simulink model "A320_Model_v1_4_3"  (R2016b)
settings: Solver=ode4  StartTime=0.0  StopTime=500  FixedStep=0.01  RelTol=1e-3
values from neighbouring files (symbols this model uses):
  er_enable = 0    [Initialization_v1_4_3.m]
  Initial_angular_rates = [0 0 0]    [Initialization_v1_4_3.m]
  initial_euler_angles = [Euler_roll_init Euler_pitch_init Euler_yaw_init]*180/pi    [Initialization_v1_4_3.m]
  initial_mulh = [41.108891 29.021111 9000]    [Initialization_v1_4_3.m]
  initial_vel_NED = transpose(DCM_init)*[U_init ; V_init ; W_init]    [Initialization_v1_4_3.m]
  tr_enable = 0    [Initialization_v1_4_3.m]
  trim_enable = 1    [Initialization_v1_4_3.m]
undefined symbols (not defined in the file or in its folder): a_Earth, acc_rand_samp, acc_rand_var, act_ang_lim_1, act_ang_lim_2, act_ang_lim_3, act_ang_lim_4, act_rate_lim_1, act_rate_lim_2, act_rate_lim_3, act_rate_lim_4, aero_CD0, aero_CD_beta, aero_CD_del_e, aero_Cl_del_a, aero_CL_del_e, aero_Cl_del_r, aero_Cl_r, aero_Cm_alpha, aero_Cm_alpha_dot, aero_Cm_del_e, aero_Cm_q, aero_Cn_beta, aero_Cn_del_r, aero_Cn_r, aero_lt_alpha_flap_CD, aero_lt_alpha_flap_CL, aero_lt_alpha_for_CD, aero_lt_alpha_for_CL, aero_lt_beta_Cl0, aero_lt_beta_CY, aero_lt_beta_for_Cl0, aero_lt_beta_for_CY, aero_lt_flap_Cm0, aero_lt_flap_for_CD, aero_lt_flap_for_CL, aero_lt_flap_for_Cm0, air_density_at_surface, air_pressure_at_surface, Aircraft_initial_mass, Aircraft_mean_chord, Aircraft_referance_area, Aircraft_wingspan, del_a_trimmed, del_e_trimmed, del_f_trimmed, del_r_trimmed, del_t_trimmed, e_Earth, engine_lt_h_for_Thrust, engine_lt_h_M_Thrust, engine_lt_M_for_Thrust, engine_number, gas_constant, gyro_rand_samp, gyro_rand_var, heat_ratio, Inertial_matrix, lapse_rate, max_thrust ... (+8)
libraries: simulink x2, aerolibtransform2 x1
settings Model: Creator=Nazmi  LastModifiedBy=Nazmi

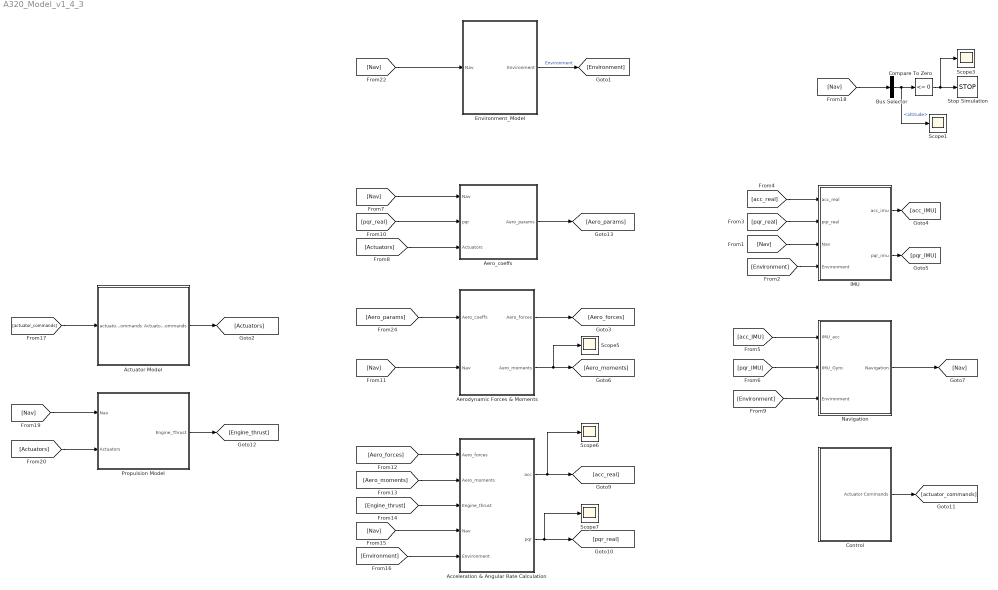
== system A320_Model_v1_4_3 ==
  Acceleration & Angular Rate Calculation : Subsystem
  Actuator Model : Subsystem
  Aero_coeffs : Subsystem
  Aerodynamic Forces & Moments : Subsystem
  Bus Selector : BusSelector  OutputSignals=mulh.altitude
  Compare To Zero : simulink/Logic and Bit Operations/Compare To Zero  relop=<=  OutDataTypeStr=boolean
  Control : Subsystem
  Environment_Model : Subsystem
  IMU : Subsystem
  Navigation : Subsystem
  "Propulsion Model " : Subsystem
  Scope{1,3,5..7} (5 alike) : Scope
  Stop Simulation : Stop
  wires:
  Navigation/1(Navigation) -> [Nav]
  [acc_IMU] -> Navigation/1(IMU_acc)
  [pqr_IMU] -> Navigation/2(IMU_Gyro)
  [Nav] -> Environment_Model/1(Nav)
  Environment_Model/1(Environment) -> [Environment]  "Environment"
  [acc_real] -> IMU/1(acc_real)
  [pqr_real] -> IMU/2(pqr_real)
  [Nav] -> IMU/3(Nav)
  [Environment] -> IMU/4(Environment)
  IMU/1(acc_imu) -> [acc_IMU]
  IMU/2(pqr_imu) -> [pqr_IMU]
  Aero_coeffs/1(Aero_params) -> [Aero_params]
  Actuator Model/1(Actuator_Commands) -> [Actuators]
  [Nav] -> Aero_coeffs/1(Nav)
  [Actuators] -> Aero_coeffs/3(Actuators)
  [Environment] -> Navigation/3(Environment)
  [pqr_real] -> Aero_coeffs/2(pqr)
  [Aero_params] -> Aerodynamic Forces & Moments/1(Aero_coeffs)
  [Nav] -> Aerodynamic Forces & Moments/2(Nav)
  Aerodynamic Forces & Moments/1(Aero_forces) -> [Aero_forces]
  Aerodynamic Forces & Moments/2(Aero_moments) -> [Aero_moments], Scope5/1
  [Aero_forces] -> Acceleration & Angular Rate Calculation/1(Aero_forces)
  [Aero_moments] -> Acceleration & Angular Rate Calculation/2(Aero_moments)
  [Engine_thrust] -> Acceleration & Angular Rate Calculation/3(Engine_thrust)
  [Nav] -> Acceleration & Angular Rate Calculation/4(Nav)
  [Environment] -> Acceleration & Angular Rate Calculation/5(Environment)
  Acceleration & Angular Rate Calculation/1(acc) -> [acc_real], Scope6/1
  Acceleration & Angular Rate Calculation/2(pqr) -> [pqr_real], Scope7/1
  Control/1(Actuator Commands) -> [actuator_commands]
  [actuator_commands] -> Actuator Model/1(actuator_commands)
  [Nav] -> Bus Selector/1
  Bus Selector/1 -> Compare To Zero/1, Scope1/1  "<altitude>"
  Compare To Zero/1 -> Stop Simulation/1, Scope3/1
  [Nav] -> "Propulsion Model "/1(Nav)
  [Actuators] -> "Propulsion Model "/2(Actuators)
  "Propulsion Model "/1("Engine_Thrust ") -> [Engine_thrust]

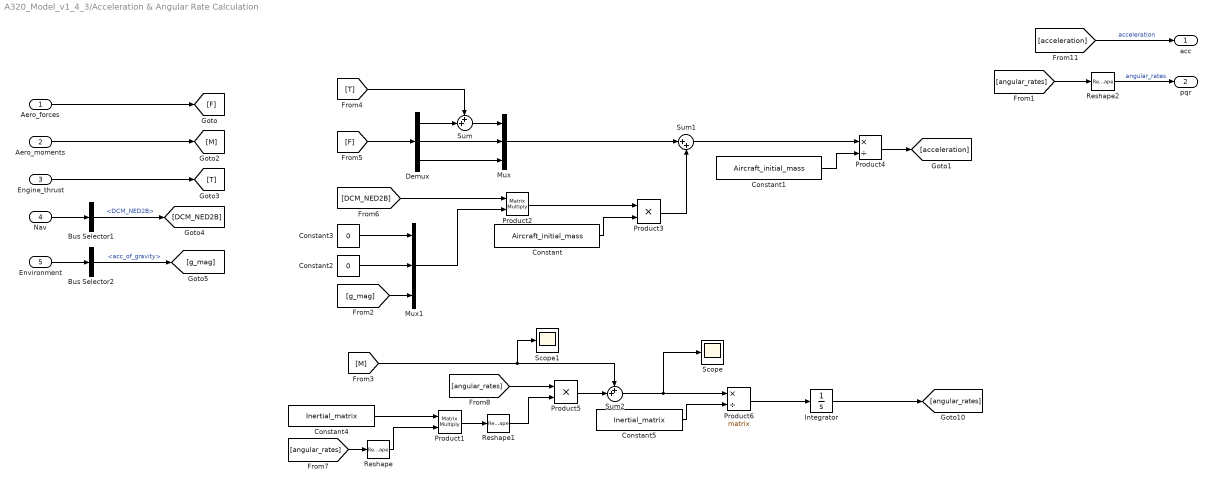
== system A320_Model_v1_4_3/Acceleration & Angular Rate Calculation ==
  Aero_forces : Inport
  Aero_moments : Inport  Port=2
  Engine_thrust : Inport  Port=3
  Nav : Inport  Port=4
  Environment : Inport  Port=5
  Bus Selector1 : BusSelector  OutputSignals=DCM_NED2B
  Bus Selector2 : BusSelector  OutputSignals=acc_of_gravity
  Constant : Constant  Value=Aircraft_initial_mass
  Constant1 : Constant  Value=Aircraft_initial_mass
  Constant2 : Constant  Value=0
  Constant3 : Constant  Value=0
  Constant4 : Constant  Value=Inertial_matrix
  Constant5 : Constant  Value=Inertial_matrix
  Demux : Demux  Outputs=3
  Integrator : Integrator  InitialCondition=Initial_angular_rates
  Mux : Mux  Inputs=3
  Mux1 : Mux  Inputs=3
  Product1 : Product  Multiplication=Matrix(*)  RndMeth=Zero
  Product2 : Product  Multiplication=Matrix(*)  RndMeth=Zero
  Product3 : Product  RndMeth=Zero
  Product4 : Product  Inputs=*/  RndMeth=Zero
  Product5 : Product  RndMeth=Zero
  Product6 : Product  Inputs=*/  Multiplication=Matrix(*)  RndMeth=Zero
  Reshape : Reshape  OutputDimensionality=Column vector (2-D)
  Reshape1 : Reshape  OutputDimensionality=Row vector (2-D)
  Reshape2 : Reshape
  Scope : Scope
  Scope1 : Scope
  Sum : Sum  Inputs=++|
  Sum1 : Sum  Inputs=|++
  Sum2 : Sum  Inputs=++|
  acc : Outport
  pqr : Outport  Port=2
  wires:
  [acceleration] -> acc/1  "acceleration"
  Aero_forces/1 -> [F]
  Aero_moments/1 -> [M]
  Engine_thrust/1 -> [T]
  Nav/1 -> Bus Selector1/1
  Environment/1 -> Bus Selector2/1
  Bus Selector1/1 -> [DCM_NED2B]  "<DCM_NED2B>"
  Bus Selector2/1 -> [g_mag]  "<acc_of_gravity>"
  Demux/1 -> Sum/2
  Sum/1 -> Mux/1
  [T] -> Sum/1
  Demux/2 -> Mux/2
  Demux/3 -> Mux/3
  [F] -> Demux/1
  [DCM_NED2B] -> Product2/1
  Product2/1 -> Product3/1
  Constant/1 -> Product3/2
  Mux/1 -> Sum1/1
  Product3/1 -> Sum1/2
  Sum1/1 -> Product4/1
  Constant1/1 -> Product4/2
  Product4/1 -> [acceleration]
  [g_mag] -> Mux1/3
  Constant3/1 -> Mux1/1
  Constant2/1 -> Mux1/2
  Mux1/1 -> Product2/2
  Product6/1 -> Integrator/1
  Constant5/1 -> Product6/2
  Sum2/1 -> Product6/1, Scope/1
  Product5/1 -> Sum2/2
  [M] -> Sum2/1, Scope1/1
  [angular_rates] -> Product5/1
  [angular_rates] -> Reshape/1
  Constant4/1 -> Product1/1
  Integrator/1 -> [angular_rates]
  Product1/1 -> Reshape1/1
  Reshape1/1 -> Product5/2
  Reshape/1 -> Product1/2
  [angular_rates] -> Reshape2/1
  Reshape2/1 -> pqr/1  "angular_rates"

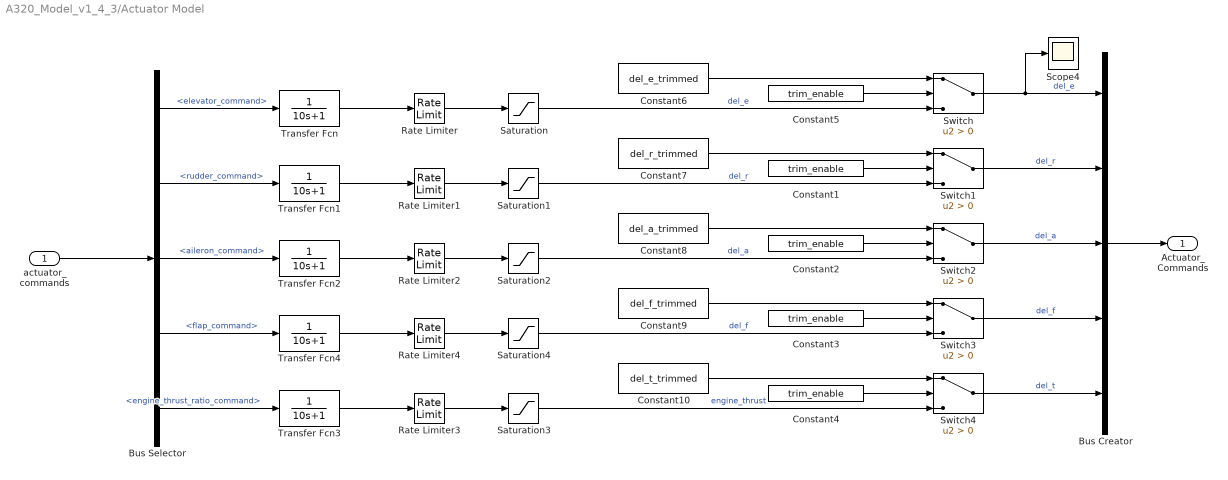
== system A320_Model_v1_4_3/Actuator Model ==
  actuator_commands : Inport
  Bus Creator : BusCreator  Inputs=5
  Bus Selector : BusSelector  OutputSignals=elevator_command,rudder_command,aileron_command,flap_command,engine_thrust_ratio_command
  Constant{1..5} (5 alike) : Constant  Value=trim_enable
  Constant10 : Constant  Value=del_t_trimmed
  Constant6 : Constant  Value=del_e_trimmed
  Constant7 : Constant  Value=del_r_trimmed
  Constant8 : Constant  Value=del_a_trimmed
  Constant9 : Constant  Value=del_f_trimmed
  Rate Limiter : RateLimiter  RisingSlewLimit=act_rate_lim_1  FallingSlewLimit=-act_rate_lim_1  SampleTimeMode=inherited
  Rate Limiter1 : RateLimiter  RisingSlewLimit=act_rate_lim_2  FallingSlewLimit=-act_rate_lim_2  SampleTimeMode=inherited
  Rate Limiter2 : RateLimiter  RisingSlewLimit=act_rate_lim_3  FallingSlewLimit=-act_rate_lim_3  SampleTimeMode=inherited
  Rate Limiter3 : RateLimiter  RisingSlewLimit=act_rate_lim_4  FallingSlewLimit=-act_rate_lim_4  SampleTimeMode=inherited
  Rate Limiter4 : RateLimiter  RisingSlewLimit=act_rate_lim_3  FallingSlewLimit=-act_rate_lim_3  SampleTimeMode=inherited
  Saturation : Saturate  UpperLimit=act_ang_lim_1  LowerLimit=-act_ang_lim_1
  Saturation1 : Saturate  UpperLimit=act_ang_lim_2  LowerLimit=-act_ang_lim_2
  Saturation2 : Saturate  UpperLimit=act_ang_lim_3  LowerLimit=-act_ang_lim_3
  Saturation3 : Saturate  UpperLimit=act_ang_lim_4  LowerLimit=0
  Saturation4 : Saturate  UpperLimit=act_ang_lim_3  LowerLimit=-act_ang_lim_3
  Scope4 : Scope
  Switch{,1..4} (5 alike) : Switch  Criteria=u2 > Threshold
  Transfer Fcn{,1..4} (5 alike) : TransferFcn  Denominator=[10 1]
  Actuator_Commands : Outport
  wires:
  Transfer Fcn/1 -> Rate Limiter/1
  Rate Limiter/1 -> Saturation/1
  Transfer Fcn1/1 -> Rate Limiter1/1
  Rate Limiter1/1 -> Saturation1/1
  Transfer Fcn2/1 -> Rate Limiter2/1
  Rate Limiter2/1 -> Saturation2/1
  Transfer Fcn3/1 -> Rate Limiter3/1
  Rate Limiter3/1 -> Saturation3/1
  Transfer Fcn4/1 -> Rate Limiter4/1
  Rate Limiter4/1 -> Saturation4/1
  Bus Creator/1 -> Actuator_Commands/1
  actuator_commands/1 -> Bus Selector/1
  Bus Selector/1 -> Transfer Fcn/1  "<elevator_command>"
  Bus Selector/2 -> Transfer Fcn1/1  "<rudder_command>"
  Bus Selector/3 -> Transfer Fcn2/1  "<aileron_command>"
  Bus Selector/4 -> Transfer Fcn4/1  "<flap_command>"
  Bus Selector/5 -> Transfer Fcn3/1  "<engine_thrust_ratio_command>"
  Saturation/1 -> Switch/3  "del_e"
  Saturation1/1 -> Switch1/3  "del_r"
  Saturation2/1 -> Switch2/3  "del_a"
  Saturation4/1 -> Switch3/3  "del_f"
  Saturation3/1 -> Switch4/3  "engine_thrust"
  Switch4/1 -> Bus Creator/5  "del_t"
  Switch2/1 -> Bus Creator/3  "del_a"
  Switch/1 -> Scope4/1, Bus Creator/1  "del_e"
  Switch1/1 -> Bus Creator/2  "del_r"
  Switch3/1 -> Bus Creator/4  "del_f"
  Constant5/1 -> Switch/2
  Constant6/1 -> Switch/1
  Constant8/1 -> Switch2/1
  Constant7/1 -> Switch1/1
  Constant9/1 -> Switch3/1
  Constant10/1 -> Switch4/1
  Constant4/1 -> Switch4/2
  Constant3/1 -> Switch3/2
  Constant2/1 -> Switch2/2
  Constant1/1 -> Switch1/2

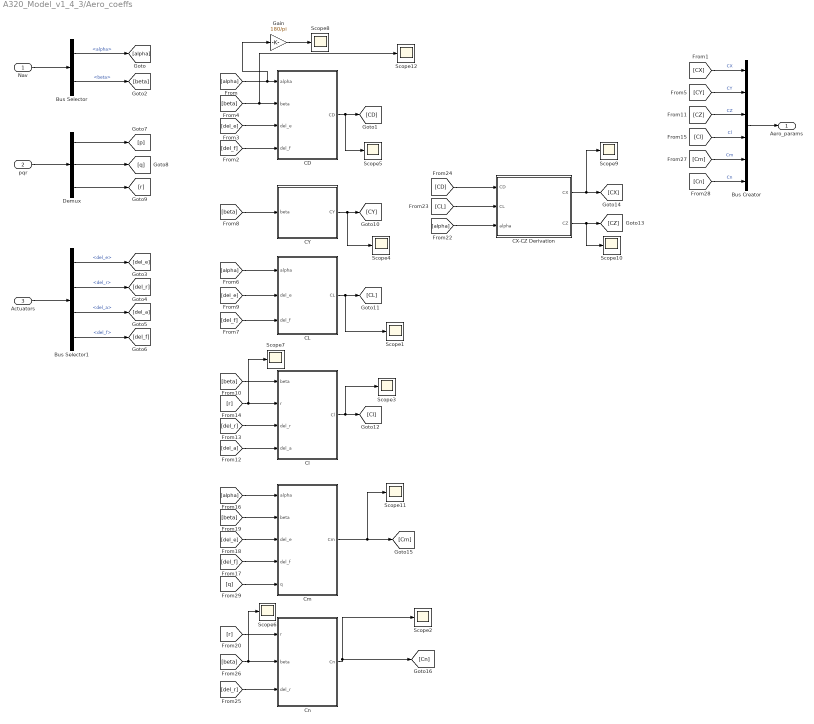
== system A320_Model_v1_4_3/Aero_coeffs ==
  Nav : Inport
  pqr : Inport  Port=2
  Actuators : Inport  Port=3
  Bus Creator : BusCreator  Inputs=6
  Bus Selector : BusSelector  OutputSignals=Flight_Performance.alpha,Flight_Performance.beta
  Bus Selector1 : BusSelector  OutputSignals=del_e,del_r,del_a,del_f
  CD : Subsystem
  CL : Subsystem
  CX-CZ Derivation : Subsystem
  CY : Subsystem
  Cl : Subsystem
  Cm : Subsystem
  Cn : Subsystem
  Demux : Demux  Outputs=3
  Gain : Gain  Gain=180/pi
  Scope{1..12} (12 alike) : Scope
  Aero_params : Outport
  wires:
  [q] -> Cm/5(q)
  [Cn] -> Bus Creator/6  "Cn"
  [Cm] -> Bus Creator/5  "Cm"
  Cn/1(Cn) -> Scope2/1, [Cn]
  [del_r] -> Cn/3(del_r)
  [beta] -> Cn/2(beta), Scope6/1
  [del_f] -> Cm/4(del_f)
  [del_e] -> Cm/3(del_e)
  [beta] -> Cm/2(beta)
  [alpha] -> Cm/1(alpha)
  [alpha] -> CX-CZ Derivation/3(alpha)
  [CL] -> CX-CZ Derivation/2(CL)
  [CD] -> CX-CZ Derivation/1(CD)
  CX-CZ Derivation/1(CX) -> [CX], Scope9/1
  CX-CZ Derivation/2(CZ) -> [CZ], Scope10/1
  [Cl] -> Bus Creator/4  "Cl"
  [del_a] -> Cl/4(del_a)
  [del_r] -> Cl/3(del_r)
  [r] -> Cl/2(r), Scope7/1
  [beta] -> Cl/1(beta)
  [CZ] -> Bus Creator/3  "CZ"
  CL/1(CL) -> [CL], Scope1/1
  [del_f] -> CL/3(del_f)
  [del_e] -> CL/2(del_e)
  [alpha] -> CL/1(alpha)
  [CY] -> Bus Creator/2  "CY"
  CY/1(CY) -> [CY], Scope4/1
  [beta] -> CY/1(beta)
  [CX] -> Bus Creator/1  "CX"
  Bus Creator/1 -> Aero_params/1
  CD/1(CD) -> [CD], Scope5/1
  [del_f] -> CD/4(del_f)
  [del_e] -> CD/3(del_e)
  [beta] -> CD/2(beta), Scope12/1
  [alpha] -> CD/1(alpha), Gain/1
  Bus Selector/2 -> [beta]  "<beta>"
  Bus Selector/1 -> [alpha]  "<alpha>"
  Nav/1 -> Bus Selector/1
  Actuators/1 -> Bus Selector1/1
  Bus Selector1/1 -> [del_e]  "<del_e>"
  Bus Selector1/2 -> [del_r]  "<del_r>"
  Bus Selector1/3 -> [del_a]  "<del_a>"
  Bus Selector1/4 -> [del_f]  "<del_f>"
  pqr/1 -> Demux/1
  Demux/1 -> [p]
  Demux/2 -> [q]
  Demux/3 -> [r]
  Cm/1(Cm) -> Scope11/1, [Cm]
  Gain/1 -> Scope8/1
  Cl/1(Cl) -> [Cl], Scope3/1
  [r] -> Cn/1(r)

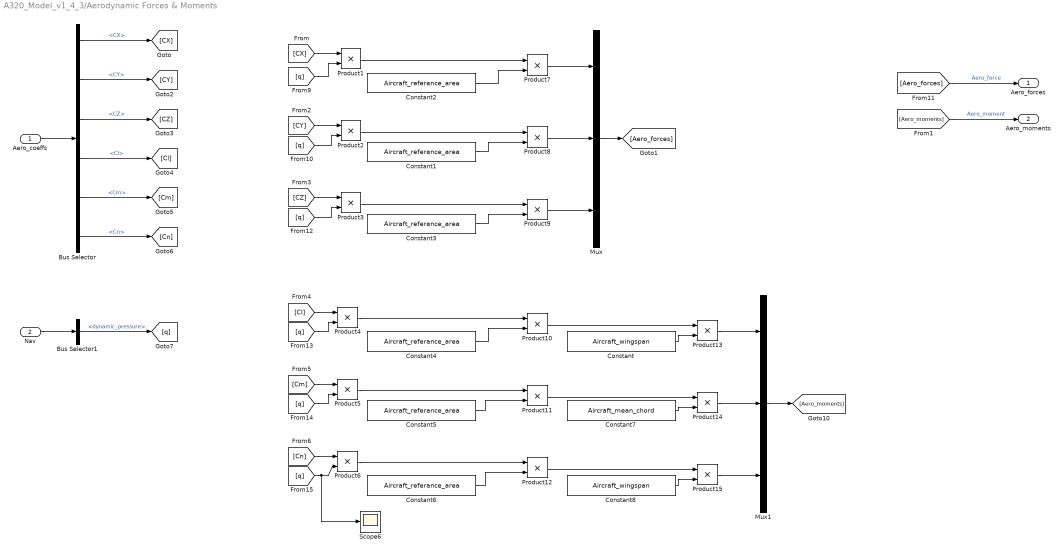
== system A320_Model_v1_4_3/Aerodynamic Forces & Moments ==
  Aero_coeffs : Inport
  Nav : Inport  Port=2
  Bus Selector : BusSelector  OutputSignals=CX,CY,CZ,Cl,Cm,Cn
  Bus Selector1 : BusSelector  OutputSignals=Flight_Performance.dynamic_pressure
  Constant : Constant  Value=Aircraft_wingspan
  Constant{1..6} (6 alike) : Constant  Value=Aircraft_referance_area
  Constant7 : Constant  Value=Aircraft_mean_chord
  Constant8 : Constant  Value=Aircraft_wingspan
  Mux : Mux  Inputs=3
  Mux1 : Mux  Inputs=3
  Product{1..15} (15 alike) : Product  RndMeth=Zero
  Scope6 : Scope
  Aero_forces : Outport
  Aero_moments : Outport  Port=2
  wires:
  Mux1/1 -> [Aero_moments]
  Mux/1 -> [Aero_forces]
  Product9/1 -> Mux/3
  Product8/1 -> Mux/2
  Product7/1 -> Mux/1
  Product15/1 -> Mux1/3
  Product14/1 -> Mux1/2
  Product13/1 -> Mux1/1
  Constant2/1 -> Product7/2
  Constant8/1 -> Product15/2
  Constant7/1 -> Product14/2
  Constant/1 -> Product13/2
  Product12/1 -> Product15/1
  Product11/1 -> Product14/1
  Product10/1 -> Product13/1
  Constant6/1 -> Product12/2
  Product6/1 -> Product12/1
  Constant5/1 -> Product11/2
  Product5/1 -> Product11/1
  Constant4/1 -> Product10/2
  Product4/1 -> Product10/1
  Constant3/1 -> Product9/2
  Product3/1 -> Product9/1
  Constant1/1 -> Product8/2
  Product2/1 -> Product8/1
  Product1/1 -> Product7/1
  [q] -> Product6/2, Scope6/1
  [Cn] -> Product6/1
  [q] -> Product5/2
  [Cm] -> Product5/1
  [q] -> Product4/2
  [Cl] -> Product4/1
  [q] -> Product3/2
  [CZ] -> Product3/1
  [q] -> Product2/2
  [CY] -> Product2/1
  [q] -> Product1/2
  [CX] -> Product1/1
  Bus Selector1/1 -> [q]  "<dynamic_pressure>"
  Nav/1 -> Bus Selector1/1
  Bus Selector/6 -> [Cn]  "<Cn>"
  Bus Selector/5 -> [Cm]  "<Cm>"
  Bus Selector/4 -> [Cl]  "<Cl>"
  Bus Selector/3 -> [CZ]  "<CZ>"
  Bus Selector/2 -> [CY]  "<CY>"
  Bus Selector/1 -> [CX]  "<CX>"
  [Aero_moments] -> Aero_moments/1  "Aero_moment"
  [Aero_forces] -> Aero_forces/1  "Aero_force"
  Aero_coeffs/1 -> Bus Selector/1

== system A320_Model_v1_4_3/Control ==
  Bus Creator2 : BusCreator  Inputs=5
  Constant{,1..4} (5 alike) : Constant  Value=0
  Actuator Commands : Outport
  wires:
  Bus Creator2/1 -> Actuator Commands/1
  Constant/1 -> Bus Creator2/1  "elevator_command"
  Constant1/1 -> Bus Creator2/2  "rudder_command"
  Constant2/1 -> Bus Creator2/3  "aileron_command"
  Constant3/1 -> Bus Creator2/4  "flap_command"
  Constant4/1 -> Bus Creator2/5  "engine_thrust_ratio_command"

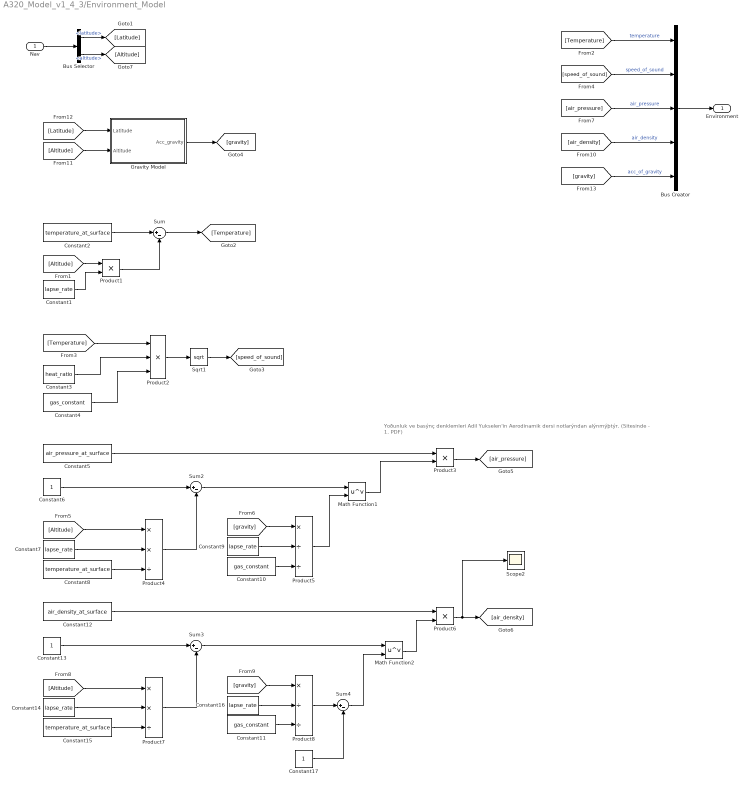
== system A320_Model_v1_4_3/Environment_Model ==
  note: Yoðunluk ve basýnç denklemleri Adil Yukselen'in Aerodinamik dersi notlarýndan alýnmýþtýr. (Sitesinde - 1. PDF)
  Nav : Inport
  Bus Creator : BusCreator  Inputs=5
  Bus Selector : BusSelector  OutputSignals=mulh.latitude,mulh.altitude
  Constant{1,7,9,14,16} (5 alike) : Constant  Value=lapse_rate
  Constant10 : Constant  Value=gas_constant
  Constant11 : Constant  Value=gas_constant
  Constant12 : Constant  Value=air_density_at_surface
  Constant13 : Constant
  Constant15 : Constant  Value=temperature_at_surface
  Constant17 : Constant
  Constant2 : Constant  Value=temperature_at_surface
  Constant3 : Constant  Value=heat_ratio
  Constant4 : Constant  Value=gas_constant
  Constant5 : Constant  Value=air_pressure_at_surface
  Constant6 : Constant
  Constant8 : Constant  Value=temperature_at_surface
  Gravity Model : Subsystem
  Math Function1 : Math  Operator=pow  SaturateOnIntegerOverflow=on
  Math Function2 : Math  Operator=pow  SaturateOnIntegerOverflow=on
  Product1 : Product  RndMeth=Zero
  Product2 : Product  Inputs=3  RndMeth=Zero
  Product3 : Product  RndMeth=Zero
  Product4 : Product  Inputs=**/  RndMeth=Zero
  Product5 : Product  Inputs=*//  RndMeth=Zero
  Product6 : Product  RndMeth=Zero
  Product7 : Product  Inputs=**/  RndMeth=Zero
  Product8 : Product  Inputs=*//  RndMeth=Zero
  Scope2 : Scope
  Sqrt1 : Sqrt  SaturateOnIntegerOverflow=on
  Sum{,2..4} (4 alike) : Sum  Inputs=|+-
  Environment : Outport
  wires:
  Nav/1 -> Bus Selector/1
  [Altitude] -> Product1/1
  Constant1/1 -> Product1/2
  Constant2/1 -> Sum/1
  Product1/1 -> Sum/2
  Sum/1 -> [Temperature]
  [Temperature] -> Bus Creator/1  "temperature"
  [Temperature] -> Product2/1
  Constant3/1 -> Product2/2
  Constant4/1 -> Product2/3
  Product2/1 -> Sqrt1/1
  Sqrt1/1 -> [speed_of_sound]
  [speed_of_sound] -> Bus Creator/2  "speed_of_sound"
  Constant5/1 -> Product3/1
  Constant6/1 -> Sum2/1
  [Altitude] -> Product4/1
  Constant7/1 -> Product4/2
  Constant8/1 -> Product4/3
  Product4/1 -> Sum2/2
  Sum2/1 -> Math Function1/1
  [gravity] -> Product5/1
  Constant9/1 -> Product5/2
  Constant10/1 -> Product5/3
  Product5/1 -> Math Function1/2
  Math Function1/1 -> Product3/2
  Product3/1 -> [air_pressure]
  [air_pressure] -> Bus Creator/3  "air_pressure"
  Constant12/1 -> Product6/1
  Constant13/1 -> Sum3/1
  [Altitude] -> Product7/1
  Constant14/1 -> Product7/2
  Constant15/1 -> Product7/3
  Product7/1 -> Sum3/2
  Sum3/1 -> Math Function2/1
  [gravity] -> Product8/1
  Constant16/1 -> Product8/2
  Constant11/1 -> Product8/3
  Math Function2/1 -> Product6/2
  Product6/1 -> [air_density], Scope2/1
  [air_density] -> Bus Creator/4  "air_density"
  Product8/1 -> Sum4/1
  Constant17/1 -> Sum4/2
  Sum4/1 -> Math Function2/2
  Gravity Model/1(Acc_gravity) -> [gravity]
  Bus Selector/1 -> [Latitude]  "<latitude>"
  Bus Selector/2 -> [Altitude]  "<altitude>"
  [Latitude] -> Gravity Model/1(Latitude)
  [Altitude] -> Gravity Model/2(Altitude)
  [gravity] -> Bus Creator/5  "acc_of_gravity"
  Bus Creator/1 -> Environment/1

== system A320_Model_v1_4_3/IMU ==
  acc_real : Inport
  pqr_real : Inport  Port=2
  Nav : Inport  Port=3
  Environment : Inport  Port=4
  Accelerometer : Subsystem
  Bus Selector : BusSelector  OutputSignals=DCM_NED2B
  Bus Selector1 : BusSelector  OutputSignals=acc_of_gravity
  Gyroscope : Subsystem
  acc_imu : Outport
  pqr_imu : Outport  Port=2
  wires:
  pqr_real/1 -> [pqr_real]
  acc_real/1 -> [acc_real]
  [acc_imu] -> acc_imu/1
  [pqr_imu] -> pqr_imu/1
  Nav/1 -> Bus Selector/1
  Bus Selector/1 -> [DCM_NED2B]  "<DCM_NED2B>"
  Accelerometer/1(acc_IMU) -> [acc_imu]
  Gyroscope/1(pqr_IMU) -> [pqr_imu]
  Environment/1 -> Bus Selector1/1
  Bus Selector1/1 -> [gravity_mag]  "<acc_of_gravity>"
  [acc_real] -> Accelerometer/1(acc_real)
  [DCM_NED2B] -> Accelerometer/2(DCM_NED2B)
  [gravity_mag] -> Accelerometer/3(g_mag)
  [pqr_real] -> Gyroscope/1(pqr_real)

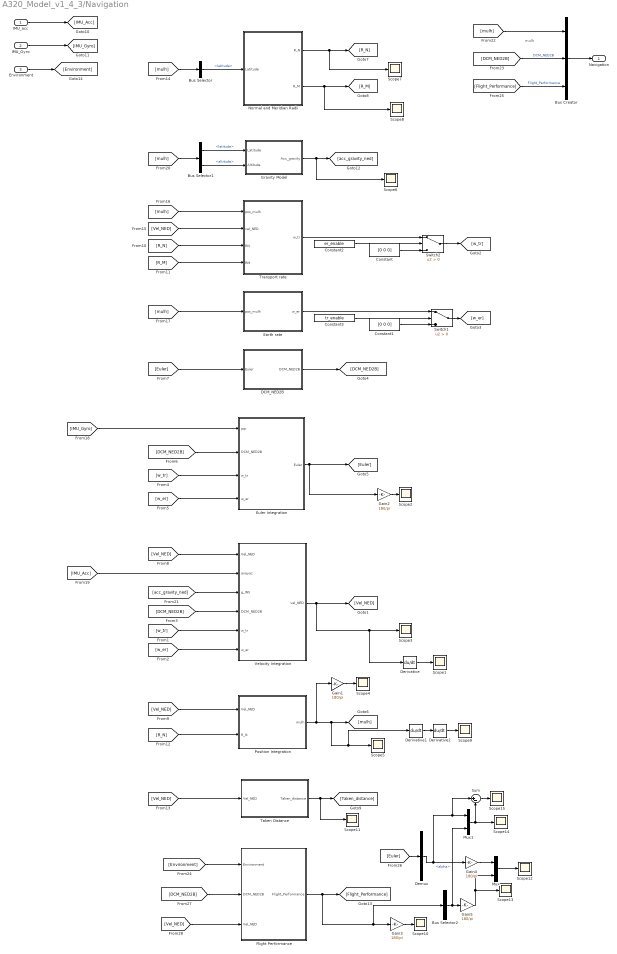
== system A320_Model_v1_4_3/Navigation ==
  note: mulh
  IMU_acc : Inport
  IMU_Gyro : Inport  Port=2
  Environment : Inport  Port=3
  Bus Creator : BusCreator  Inputs=3
  Bus Selector : BusSelector  OutputSignals=latitude
  Bus Selector1 : BusSelector  OutputSignals=latitude,altitude
  Bus Selector2 : BusSelector  OutputSignals=alpha
  Constant : Constant  Value=[0 0 0]
  Constant1 : Constant  Value=[0 0 0]
  Constant2 : Constant  Value=er_enable
  Constant3 : Constant  Value=tr_enable
  DCM_NED2B : Subsystem
  Demux : Demux  Outputs=3
  Derivative : Derivative
  Derivative1 : Derivative
  Derivative2 : Derivative
  Earth rate : Subsystem
  Euler Integration : Subsystem
  Flight Performance : Subsystem
  Gain{1..5} (5 alike) : Gain  Gain=180/pi
  Gravity Model : Subsystem
  Mux : Mux  Inputs=2
  Mux1 : Mux  Inputs=2
  Normal and Meridian Radii : Subsystem
  Position Integration : Subsystem
  Scope{1..15} (15 alike) : Scope
  Sum : Sum  Inputs=|+-
  Switch1 : Switch  Criteria=u2 > Threshold
  Switch2 : Switch  Criteria=u2 > Threshold
  Taken Distance : Subsystem
  Transport rate : Subsystem
  Velocity Integration : Subsystem
  Navigation : Outport
  wires:
  Normal and Meridian Radii/1(R_N) -> [R_N], Scope7/1
  Normal and Meridian Radii/2(R_M) -> [R_M], Scope8/1
  [mulh] -> Transport rate/1(pos_mulh)
  [Vel_NED] -> Transport rate/2(vel_NED)
  Transport rate/1(w_tr) -> Switch2/1
  [Euler] -> DCM_NED2B/1(Euler)
  DCM_NED2B/1(DCM_NED2B) -> [DCM_NED2B]
  [IMU_Gyro] -> Euler Integration/1(pqr)
  Gain2/1 -> Scope2/1
  Euler Integration/1(Euler) -> [Euler], Gain2/1
  [DCM_NED2B] -> Euler Integration/2(DCM_NED2B)
  [w_tr] -> Euler Integration/3(w_tr)
  [w_er] -> Euler Integration/4(w_er)
  [IMU_Acc] -> Velocity Integration/2(axayaz)
  [DCM_NED2B] -> Velocity Integration/4(DCM_NED2B)
  [w_tr] -> Velocity Integration/5(w_tr)
  [w_er] -> Velocity Integration/6(w_er)
  [acc_gravity_ned] -> Velocity Integration/3(g_INS)
  Velocity Integration/1(vel_NED) -> Scope3/1, Derivative/1, [Vel_NED]
  [Vel_NED] -> Velocity Integration/1(Vel_NED)
  [Vel_NED] -> Position Integration/1(Vel_NED)
  Position Integration/1(mulh) -> [mulh], Scope5/1, Derivative1/1, Gain1/1
  [R_N] -> Transport rate/3(RN)
  [R_M] -> Transport rate/4(RM)
  [R_N] -> Position Integration/2(R_N)
  [mulh] -> Bus Selector/1
  Bus Selector/1 -> Normal and Meridian Radii/1(Latitude)  "<latitude>"
  [mulh] -> Earth rate/1(pos_mulh)
  Derivative/1 -> Scope1/1
  Gain1/1 -> Scope4/1
  Derivative1/1 -> Derivative2/1
  Derivative2/1 -> Scope9/1
  [Vel_NED] -> Taken Distance/1(Vel_NED)
  Taken Distance/1(Taken_distance) -> [Taken_distance], Scope11/1
  [mulh] -> Bus Selector1/1
  Bus Selector1/1 -> Gravity Model/1(Latitude)  "<latitude>"
  Bus Selector1/2 -> Gravity Model/2(Altitude)  "<altitude>"
  Gravity Model/1(Acc_gravity) -> [acc_gravity_ned], Scope6/1
  IMU_acc/1 -> [IMU_Acc]
  IMU_Gyro/1 -> [IMU_Gyro]
  [mulh] -> Bus Creator/1
  Bus Creator/1 -> Navigation/1
  [DCM_NED2B] -> Bus Creator/2  "DCM_NED2B"
  Gain3/1 -> Scope10/1
  Flight Performance/1(Flight_Performance) -> [Flight_Performance], Gain3/1, Bus Selector2/1
  [DCM_NED2B] -> Flight Performance/2(DCM_NED2B)
  [Vel_NED] -> Flight Performance/3(Vel_NED)
  [Environment] -> Flight Performance/1(Environment)
  Environment/1 -> [Environment]
  [Flight_Performance] -> Bus Creator/3  "Flight_Performance"
  Gain4/1 -> Mux/1
  [Euler] -> Demux/1
  Bus Selector2/1 -> Gain5/1, Mux1/2  "<alpha>"
  Mux/1 -> Scope12/1
  Gain5/1 -> Mux/2, Scope13/1
  Demux/2 -> Gain4/1, Mux1/1, Sum/1
  Mux1/1 -> Scope14/1, Sum/2
  Sum/1 -> Scope15/1
  Switch2/1 -> [w_tr]
  Constant/1 -> Switch2/3
  Switch1/1 -> [w_er]
  Earth rate/1(w_er) -> Switch1/1
  Constant3/1 -> Switch1/2
  Constant1/1 -> Switch1/3
  Constant2/1 -> Switch2/2

== system A320_Model_v1_4_3/Propulsion Model  ==
  Nav : Inport
  Actuators : Inport  Port=2
  2-D Lookup Table : Lookup_n-D  BreakpointsForDimension1=engine_lt_M_for_Thrust  BreakpointsForDimension2=engine_lt_h_for_Thrust  Table=engine_lt_h_M_Thrust  RndMeth=Simplest  InputSameDT=on
  Bus Selector : BusSelector  OutputSignals=mulh.altitude,Flight_Performance.Mach
  Bus Selector1 : BusSelector  OutputSignals=del_t
  Constant10 : Constant  Value=10000
  Max Thrust : Constant  Value=max_thrust
  "Number of Engines " : Constant  Value=engine_number
  Product : Product
  Product1 : Product  Inputs=3
  "Engine_Thrust " : Outport
  wires:
  Nav/1 -> Bus Selector/1
  Bus Selector/1 -> [Altitude]  "<altitude>"
  "Number of Engines "/1 -> Product/2
  Max Thrust/1 -> Product/1
  [Altitude] -> 2-D Lookup Table/2
  [Mach] -> 2-D Lookup Table/1
  Product1/1 -> [Engine_thrust]
  [Engine_thrust] -> "Engine_Thrust "/1  "Engine_Thrust"
  Bus Selector/2 -> [Mach]  "<Mach>"
  Product/1 -> Product1/2
  Actuators/1 -> Bus Selector1/1
  Bus Selector1/1 -> [del_t]  "<del_t>"
  2-D Lookup Table/1 -> Product1/1
  [del_t] -> Product1/3

== system A320_Model_v1_4_3/Aero_coeffs/CD ==
  alpha : Inport
  beta : Inport  Port=2
  del_e : Inport  Port=3
  del_f : Inport  Port=4
  2-D Lookup Table1 : Lookup_n-D  BreakpointsForDimension1=aero_lt_alpha_for_CD  BreakpointsForDimension2=aero_lt_flap_for_CD  Table=aero_lt_alpha_flap_CD  RndMeth=Simplest  InputSameDT=on
  Abs : Abs
  Abs1 : Abs
  Add : Sum  Inputs=4
  Constant : Constant  Value=aero_CD0
  Constant1 : Constant  Value=aero_CD_del_e
  Constant2 : Constant  Value=aero_CD_beta
  Product1 : Product  RndMeth=Zero
  Product2 : Product  RndMeth=Zero
  Scope2 : Scope
  Scope3 : Scope
  Scope5 : Scope
  CD : Outport
  wires:
  Abs1/1 -> Product2/2
  Abs/1 -> Product1/2
  Add/1 -> CD/1
  Product2/1 -> Add/4, Scope3/1
  Product1/1 -> Add/3, Scope2/1
  Constant/1 -> Scope5/1, Add/1
  [beta] -> Abs1/1
  Constant2/1 -> Product2/1
  [del_e] -> Abs/1
  Constant1/1 -> Product1/1
  2-D Lookup Table1/1 -> Add/2
  [del_f] -> 2-D Lookup Table1/2
  [alpha] -> 2-D Lookup Table1/1
  del_f/1 -> [del_f]
  del_e/1 -> [del_e]
  beta/1 -> [beta]
  alpha/1 -> [alpha]

== system A320_Model_v1_4_3/Aero_coeffs/CL ==
  alpha : Inport
  del_e : Inport  Port=2
  del_f : Inport  Port=3
  2-D Lookup Table1 : Lookup_n-D  BreakpointsForDimension1=aero_lt_alpha_for_CL  BreakpointsForDimension2=aero_lt_flap_for_CL  Table=aero_lt_alpha_flap_CL  RndMeth=Simplest  InputSameDT=on
  Add : Sum  Inputs=2
  Constant1 : Constant  Value=aero_CL_del_e
  Product1 : Product  RndMeth=Zero
  Scope1 : Scope
  Scope2 : Scope
  Scope5 : Scope
  CL : Outport
  wires:
  alpha/1 -> [alpha]
  del_e/1 -> [del_e]
  del_f/1 -> [del_f]
  [alpha] -> 2-D Lookup Table1/1
  [del_f] -> 2-D Lookup Table1/2
  Constant1/1 -> Product1/1
  [del_e] -> Product1/2
  Add/1 -> CL/1, Scope2/1
  2-D Lookup Table1/1 -> Add/1, Scope5/1
  Product1/1 -> Add/2, Scope1/1

== system A320_Model_v1_4_3/Aero_coeffs/CX-CZ Derivation ==
  CD : Inport
  CL : Inport  Port=2
  alpha : Inport  Port=3
  Gain : Gain  Gain=-1
  Gain1 : Gain  Gain=-1
  Product{,1..3} (4 alike) : Product  RndMeth=Zero
  Sum : Sum  Inputs=|++
  Sum1 : Sum  Inputs=|+-
  Trigonometric Function1 : Trigonometry  Operator=cos
  Trigonometric Function2 : Trigonometry
  Trigonometric Function3 : Trigonometry
  Trigonometric Function4 : Trigonometry  Operator=cos
  CX : Outport
  CZ : Outport  Port=2
  wires:
  Sum/1 -> Gain/1
  alpha/1 -> [alpha]
  CL/1 -> [CL]
  Sum1/1 -> Gain1/1
  CD/1 -> [CD]
  Product2/1 -> Sum1/2
  Product3/1 -> Sum1/1
  [CD] -> Product3/2
  Trigonometric Function4/1 -> Product3/1
  [alpha] -> Trigonometric Function4/1
  [CL] -> Product2/2
  Trigonometric Function3/1 -> Product2/1
  [alpha] -> Trigonometric Function3/1
  Product/1 -> Sum/2
  Product1/1 -> Sum/1
  [CD] -> Product1/2
  Trigonometric Function2/1 -> Product1/1
  [alpha] -> Trigonometric Function2/1
  [CL] -> Product/2
  Trigonometric Function1/1 -> Product/1
  [alpha] -> Trigonometric Function1/1
  Gain/1 -> CZ/1
  Gain1/1 -> CX/1

== system A320_Model_v1_4_3/Aero_coeffs/CY ==
  beta : Inport
  1-D Lookup Table : Lookup_n-D  NumberOfTableDimensions=1  BreakpointsForDimension1=aero_lt_beta_for_CY  Table=aero_lt_beta_CY  RndMeth=Simplest  InputSameDT=on
  Product1 : Product  RndMeth=Zero
  Scope5 : Scope
  CY : Outport
  wires:
  [beta] -> Product1/2, 1-D Lookup Table/1
  Product1/1 -> CY/1, Scope5/1
  beta/1 -> [beta]
  1-D Lookup Table/1 -> Product1/1

== system A320_Model_v1_4_3/Aero_coeffs/Cl ==
  beta : Inport
  r : Inport  Port=2
  del_r : Inport  Port=3
  del_a : Inport  Port=4
  1-D Lookup Table : Lookup_n-D  NumberOfTableDimensions=1  BreakpointsForDimension1=aero_lt_beta_for_Cl0  Table=aero_lt_beta_Cl0  RndMeth=Simplest  InputSameDT=on
  Add : Sum  Inputs=4
  Constant1 : Constant  Value=aero_Cl_del_r
  Constant2 : Constant  Value=aero_Cl_del_a
  Constant3 : Constant  Value=aero_Cl_r
  Product{,1..3} (4 alike) : Product  RndMeth=Zero
  Scope{1..4} (4 alike) : Scope
  Cl : Outport
  wires:
  [beta] -> Product3/2, 1-D Lookup Table/1
  1-D Lookup Table/1 -> Product3/1
  Product3/1 -> Add/1, Scope3/1
  [del_a] -> Product2/2
  [del_r] -> Product1/2
  Constant3/1 -> Product/1
  beta/1 -> [beta]
  r/1 -> [r]
  del_r/1 -> [del_r]
  del_a/1 -> [del_a]
  [r] -> Product/2
  Constant1/1 -> Product1/1
  Constant2/1 -> Product2/1
  Product/1 -> Add/2, Scope4/1
  Product1/1 -> Add/3, Scope2/1
  Product2/1 -> Add/4, Scope1/1
  Add/1 -> Cl/1

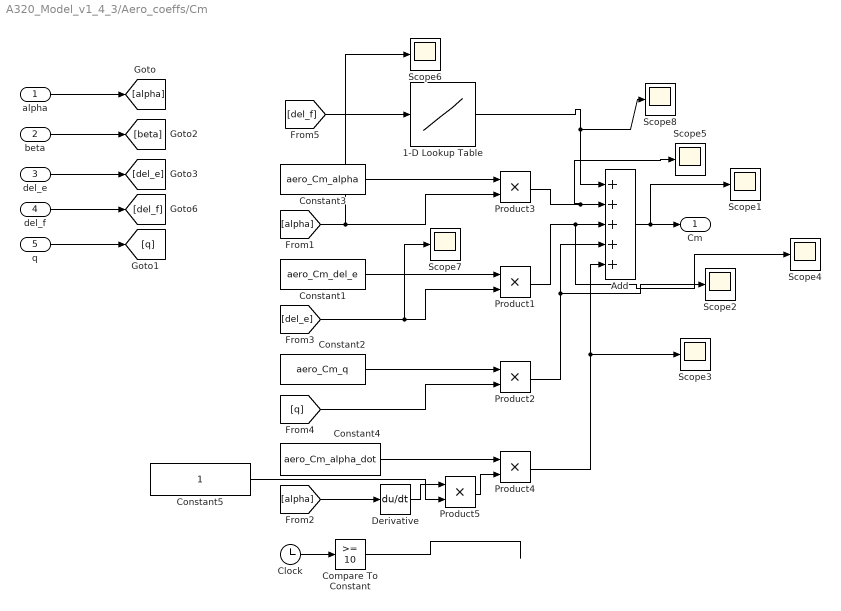
== system A320_Model_v1_4_3/Aero_coeffs/Cm ==
  alpha : Inport
  beta : Inport  Port=2
  del_e : Inport  Port=3
  del_f : Inport  Port=4
  q : Inport  Port=5
  1-D Lookup Table : Lookup_n-D  NumberOfTableDimensions=1  BreakpointsForDimension1=aero_lt_flap_for_Cm0  Table=aero_lt_flap_Cm0  RndMeth=Simplest  InputSameDT=on
  Add : Sum  Inputs=5
  Clock : Clock
  Compare To Constant : simulink/Logic and Bit Operations/Compare To Constant  relop=>=  const=10  OutDataTypeStr=uint8
  Constant1 : Constant  Value=aero_Cm_del_e
  Constant2 : Constant  Value=aero_Cm_q
  Constant3 : Constant  Value=aero_Cm_alpha
  Constant4 : Constant  Value=aero_Cm_alpha_dot
  Constant5 : Constant
  Derivative : Derivative
  Product{1..5} (5 alike) : Product  RndMeth=Zero
  Scope{1..8} (8 alike) : Scope
  Cm : Outport
  wires:
  Product4/1 -> Add/5, Scope3/1
  Constant4/1 -> Product4/1
  Product2/1 -> Add/4, Scope2/1
  q/1 -> [q]
  [alpha] -> Derivative/1
  [alpha] -> Product3/2, Scope6/1
  Constant3/1 -> Product3/1
  Add/1 -> Scope1/1, Cm/1
  Product1/1 -> Add/3, Scope4/1
  Product3/1 -> Scope5/1, Add/2
  [del_f] -> 1-D Lookup Table/1
  [q] -> Product2/2
  Constant2/1 -> Product2/1
  [del_e] -> Scope7/1, Product1/2
  Constant1/1 -> Product1/1
  del_f/1 -> [del_f]
  del_e/1 -> [del_e]
  beta/1 -> [beta]
  alpha/1 -> [alpha]
  1-D Lookup Table/1 -> Scope8/1, Add/1
  Product5/1 -> Product4/2
  Derivative/1 -> Product5/1
  Compare To Constant/1 -> ?
  Clock/1 -> Compare To Constant/1
  Constant5/1 -> Product5/2

== system A320_Model_v1_4_3/Aero_coeffs/Cn ==
  r : Inport
  beta : Inport  Port=2
  del_r : Inport  Port=3
  Add : Sum  Inputs=3
  Constant1 : Constant  Value=aero_Cn_beta
  Constant2 : Constant  Value=aero_Cn_del_r
  Constant3 : Constant  Value=aero_Cn_r
  Product1 : Product  RndMeth=Zero
  Product2 : Product  RndMeth=Zero
  Product3 : Product  RndMeth=Zero
  Scope{1..4} (4 alike) : Scope
  Cn : Outport
  wires:
  Product2/1 -> Add/3, Scope3/1
  Product1/1 -> Add/2, Scope1/1
  Product3/1 -> Add/1, Scope2/1
  [r] -> Product3/2
  Constant3/1 -> Product3/1
  Add/1 -> Cn/1, Scope4/1
  [del_r] -> Product2/2
  Constant2/1 -> Product2/1
  [beta] -> Product1/2
  Constant1/1 -> Product1/1
  del_r/1 -> [del_r]
  beta/1 -> [beta]
  r/1 -> [r]

== system A320_Model_v1_4_3/Environment_Model/Gravity Model ==
  note: Somigliana denklemi uygulanmýþtýr. Noureldin-Karamat sf.53
  Latitude : Inport
  Altitude : Inport  Port=2
  Constant : Constant
  Constant2 : Constant  Value=somigliana_coeff_a2
  Constant3 : Constant  Value=somigliana_coeff_a3
  Constant4 : Constant  Value=somigliana_coeff_a1
  Constant5 : Constant  Value=somigliana_coeff_a4
  Constant6 : Constant  Value=somigliana_coeff_a5
  Constant7 : Constant  Value=somigliana_coeff_a6
  Product{,2,4..6} (5 alike) : Product  RndMeth=Zero
  Product3 : Product  Inputs=3  RndMeth=Zero
  Product7 : Product  Inputs=3  RndMeth=Zero
  Sum1 : Sum  Inputs=+++
  Sum2 : Sum  Inputs=+++
  Sum3 : Sum  Inputs=|++
  Trigonometric Function2 : Trigonometry
  Acc_gravity : Outport
  wires:
  Altitude/1 -> [Altitude]
  Latitude/1 -> Trigonometric Function2/1
  Product/1 -> [sL2]
  Trigonometric Function2/1 -> Product/1, Product/2
  Constant2/1 -> Product2/1
  [sL2] -> Product2/2
  [sL2] -> Product3/2, Product3/3
  Constant3/1 -> Product3/1
  Constant/1 -> Sum2/1
  Product2/1 -> Sum2/2
  Product3/1 -> Sum2/3
  Constant4/1 -> Product4/1
  Sum2/1 -> Product4/2
  Product4/1 -> Sum1/1
  Constant5/1 -> Sum3/1
  Constant6/1 -> Product5/1
  [sL2] -> Product5/2
  Product5/1 -> Sum3/2
  Sum3/1 -> Product6/1
  [Altitude] -> Product6/2
  Product6/1 -> Sum1/2
  Constant7/1 -> Product7/1
  [Altitude] -> Product7/2, Product7/3
  Product7/1 -> Sum1/3
  Sum1/1 -> [acc_grav]
  [acc_grav] -> Acc_gravity/1

== system A320_Model_v1_4_3/IMU/Accelerometer ==
  acc_real : Inport
  DCM_NED2B : Inport  Port=2
  g_mag : Inport  Port=3
  Demux : Demux  Outputs=3
  Math Function : Math  Operator=transpose  SaturateOnIntegerOverflow=on
  Mux : Mux  Inputs=3
  Mux1 : Mux  Inputs=3
  Product : Product  Multiplication=Matrix(*)  RndMeth=Zero
  Product1 : Product  Multiplication=Matrix(*)  RndMeth=Zero
  Random Number : RandomNumber  Variance=acc_rand_var  SampleTime=acc_rand_samp
  Random Number1 : RandomNumber  Variance=acc_rand_var  SampleTime=acc_rand_samp
  Random Number2 : RandomNumber  Variance=acc_rand_var  SampleTime=acc_rand_samp
  Sum : Sum  Inputs=|++
  Sum1 : Sum  Inputs=|+-
  acc_IMU : Outport
  wires:
  [acc_IMU] -> acc_IMU/1
  acc_real/1 -> [acc_real]
  Random Number/1 -> Mux/1
  Random Number1/1 -> Mux/2
  Random Number2/1 -> Mux/3
  Sum/1 -> [acc_IMU]
  Mux/1 -> ?
  DCM_NED2B/1 -> [DCM_NED2B]
  [DCM_NED2B] -> Math Function/1
  Math Function/1 -> Product/1
  [acc_real] -> Product/2
  Product/1 -> Demux/1
  Demux/1 -> Mux1/1
  Demux/2 -> Mux1/2
  Demux/3 -> Sum1/1
  Sum1/1 -> Mux1/3
  g_mag/1 -> [g_mag]
  [g_mag] -> Sum1/2
  [DCM_NED2B] -> Product1/1
  Mux1/1 -> Product1/2
  Product1/1 -> Sum/1

== system A320_Model_v1_4_3/IMU/Gyroscope ==
  pqr_real : Inport
  Mux : Mux  Inputs=3
  Random Number : RandomNumber  Variance=gyro_rand_var  SampleTime=gyro_rand_samp
  Random Number1 : RandomNumber  Variance=gyro_rand_var  SampleTime=gyro_rand_samp
  Random Number2 : RandomNumber  Variance=gyro_rand_var  SampleTime=gyro_rand_samp
  Sum : Sum  Inputs=|++
  pqr_IMU : Outport
  wires:
  pqr_real/1 -> [pqr_FM]
  [pqr_IMU] -> pqr_IMU/1
  Random Number/1 -> Mux/1
  Random Number1/1 -> Mux/2
  Random Number2/1 -> Mux/3
  [pqr_FM] -> Sum/1
  Sum/1 -> [pqr_IMU]
  Mux/1 -> ?

== system A320_Model_v1_4_3/Navigation/DCM_NED2B ==
  Euler : Inport
  Demux : Demux  Outputs=3
  Mux : Mux  Inputs=3
  Rotation Angles to Direction Cosine Matrix : aerolibtransform2/Rotation Angles to Direction Cosine Matrix  rotationOrder=ZYX
  DCM_NED2B : Outport
  wires:
  [DCM_NED2B] -> DCM_NED2B/1  "DCM_NED2B"
  Euler/1 -> [Euler]
  Rotation Angles to Direction Cosine Matrix/1 -> [DCM_NED2B]
  [Euler] -> Demux/1
  Mux/1 -> Rotation Angles to Direction Cosine Matrix/1
  Demux/3 -> Mux/1
  Demux/1 -> Mux/3
  Demux/2 -> Mux/2

== system A320_Model_v1_4_3/Navigation/Earth rate ==
  pos_mulh : Inport
  Constant : Constant  Value=w_Earth
  Constant1 : Constant  Value=0
  Constant2 : Constant  Value=w_Earth
  Demux : Demux  Outputs=3
  Gain2 : Gain  Gain=-1
  Mux : Mux  Inputs=3
  Product1 : Product  Inputs=**  RndMeth=Zero
  Product2 : Product  Inputs=**  RndMeth=Zero
  Terminator : Terminator
  Terminator1 : Terminator
  Trigonometric Function1 : Trigonometry  Operator=cos
  Trigonometric Function2 : Trigonometry
  w_er : Outport
  wires:
  Mux/1 -> [w_err]
  Product1/1 -> Mux/1
  pos_mulh/1 -> Demux/1
  Demux/3 -> Terminator1/1
  Demux/2 -> Terminator/1
  Demux/1 -> [lat]
  [w_err] -> w_er/1  "earth_rate"
  [lat] -> Trigonometric Function1/1
  Trigonometric Function1/1 -> Product1/1
  Constant1/1 -> Mux/2
  [lat] -> Trigonometric Function2/1
  Trigonometric Function2/1 -> Product2/1
  Constant2/1 -> Gain2/1
  Gain2/1 -> Product2/2
  Product2/1 -> Mux/3
  Constant/1 -> Product1/2

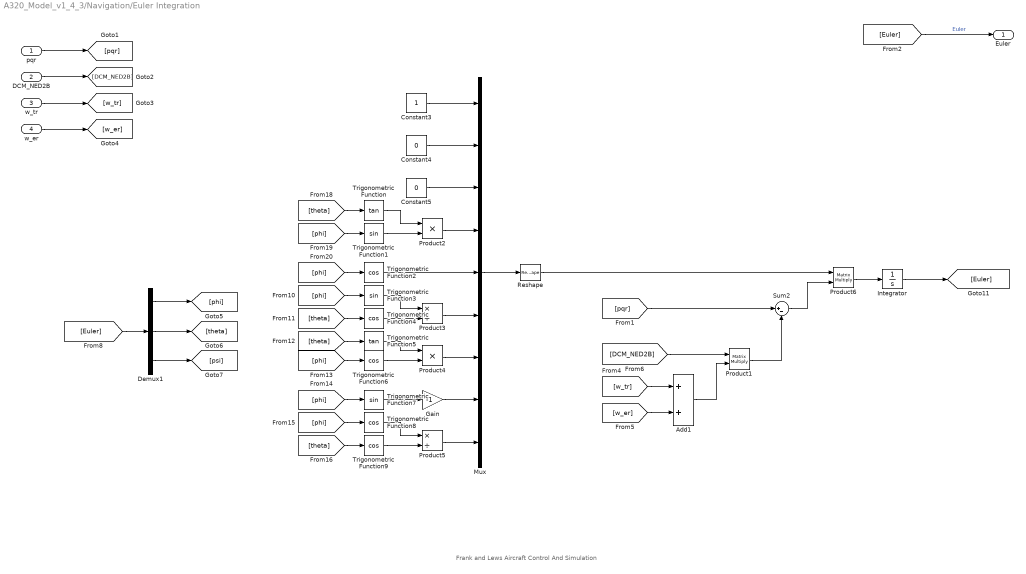
== system A320_Model_v1_4_3/Navigation/Euler Integration ==
  note: Frank and Lews Aircraft Control And Simulation
  pqr : Inport
  DCM_NED2B : Inport  Port=2
  w_tr : Inport  Port=3
  w_er : Inport  Port=4
  Add1 : Sum
  Constant3 : Constant
  Constant4 : Constant  Value=0
  Constant5 : Constant  Value=0
  Demux1 : Demux  Outputs=3
  Gain : Gain  Gain=-1
  Integrator : Integrator  InitialCondition=initial_euler_angles*pi/180
  Mux : Mux  Inputs=9
  Product1 : Product  Multiplication=Matrix(*)  RndMeth=Zero
  Product2 : Product  RndMeth=Zero
  Product3 : Product  Inputs=*/  RndMeth=Zero
  Product4 : Product  RndMeth=Zero
  Product5 : Product  Inputs=*/  RndMeth=Zero
  Product6 : Product  Multiplication=Matrix(*)  RndMeth=Zero
  Reshape : Reshape  OutputDimensionality=Customize  OutputDimensions=[3,3]
  Sum2 : Sum  Inputs=|+-
  Trigonometric Function : Trigonometry  Operator=tan
  Trigonometric Function1 : Trigonometry
  Trigonometric Function{2,4,6,8..9} (5 alike) : Trigonometry  Operator=cos
  Trigonometric Function3 : Trigonometry
  Trigonometric Function5 : Trigonometry  Operator=tan
  Trigonometric Function7 : Trigonometry
  Euler : Outport
  wires:
  Add1/1 -> Product1/2
  [pqr] -> Sum2/1
  Product1/1 -> Sum2/2
  [w_tr] -> Add1/1
  [w_er] -> Add1/2
  [DCM_NED2B] -> Product1/1
  Demux1/1 -> [phi]
  Demux1/2 -> [theta]
  Demux1/3 -> [psi]
  [Euler] -> Demux1/1
  Sum2/1 -> Product6/2
  Product6/1 -> Integrator/1
  Integrator/1 -> [Euler]
  pqr/1 -> [pqr]
  [Euler] -> Euler/1  "Euler"
  DCM_NED2B/1 -> [DCM_NED2B]
  w_tr/1 -> [w_tr]
  w_er/1 -> [w_er]
  Reshape/1 -> Product6/1
  Constant3/1 -> Mux/1
  Constant4/1 -> Mux/2
  Constant5/1 -> Mux/3
  [theta] -> Trigonometric Function/1
  [phi] -> Trigonometric Function1/1
  Product2/1 -> Mux/4
  Trigonometric Function/1 -> Product2/1
  Trigonometric Function1/1 -> Product2/2
  [phi] -> Trigonometric Function2/1
  Trigonometric Function2/1 -> Mux/5
  [theta] -> Trigonometric Function4/1
  Trigonometric Function3/1 -> Product3/1
  Trigonometric Function4/1 -> Product3/2
  Product3/1 -> Mux/6
  [phi] -> Trigonometric Function3/1
  [theta] -> Trigonometric Function5/1
  [phi] -> Trigonometric Function6/1
  Trigonometric Function5/1 -> Product4/1
  Trigonometric Function6/1 -> Product4/2
  Product4/1 -> Mux/7
  [phi] -> Trigonometric Function7/1
  Trigonometric Function7/1 -> Gain/1
  Gain/1 -> Mux/8
  [theta] -> Trigonometric Function9/1
  Trigonometric Function8/1 -> Product5/1
  Trigonometric Function9/1 -> Product5/2
  [phi] -> Trigonometric Function8/1
  Product5/1 -> Mux/9
  Mux/1 -> Reshape/1

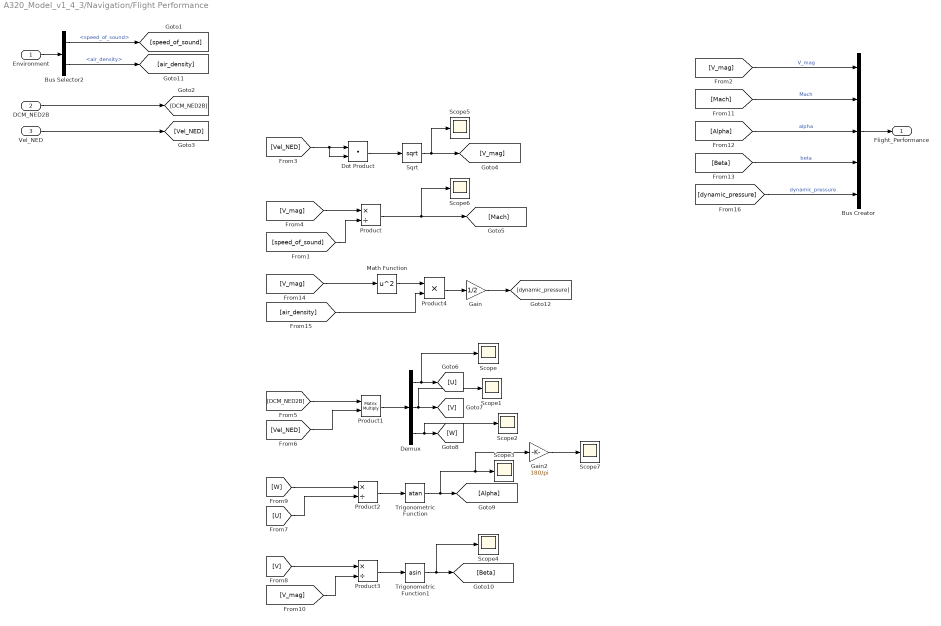
== system A320_Model_v1_4_3/Navigation/Flight Performance ==
  Environment : Inport
  DCM_NED2B : Inport  Port=2
  Vel_NED : Inport  Port=3
  Bus Creator : BusCreator  Inputs=5
  Bus Selector2 : BusSelector  OutputSignals=speed_of_sound,air_density
  Demux : Demux  Outputs=3
  Dot Product : DotProduct  InputSameDT=on  OutDataTypeStr=Inherit: Inherit via internal rule
  Gain : Gain  Gain=1/2
  Gain2 : Gain  Gain=180/pi
  Math Function : Math  Operator=square  SaturateOnIntegerOverflow=on
  Product : Product  Inputs=*/  RndMeth=Zero
  Product1 : Product  Multiplication=Matrix(*)  RndMeth=Zero
  Product2 : Product  Inputs=*/  RndMeth=Zero
  Product3 : Product  Inputs=*/  RndMeth=Zero
  Product4 : Product  RndMeth=Zero
  Scope{,1..7} (8 alike) : Scope
  Sqrt : Sqrt  SaturateOnIntegerOverflow=on
  Trigonometric Function : Trigonometry  Operator=atan
  Trigonometric Function1 : Trigonometry  Operator=asin
  Flight_Performance : Outport
  wires:
  Vel_NED/1 -> [Vel_NED]
  DCM_NED2B/1 -> [DCM_NED2B]
  Environment/1 -> Bus Selector2/1
  Bus Selector2/1 -> [speed_of_sound]  "<speed_of_sound>"
  [Vel_NED] -> Dot Product/1, Dot Product/2
  Dot Product/1 -> Sqrt/1
  Sqrt/1 -> [V_mag], Scope5/1
  [V_mag] -> Product/1
  [speed_of_sound] -> Product/2
  Product/1 -> [Mach], Scope6/1
  [DCM_NED2B] -> Product1/1
  [Vel_NED] -> Product1/2
  Product1/1 -> Demux/1
  Demux/1 -> [U], Scope/1
  Demux/2 -> [V], Scope1/1
  Demux/3 -> [W], Scope2/1
  [W] -> Product2/1
  [U] -> Product2/2
  Product2/1 -> Trigonometric Function/1
  Trigonometric Function/1 -> [Alpha], Scope3/1, Gain2/1
  [V] -> Product3/1
  [V_mag] -> Product3/2
  Product3/1 -> Trigonometric Function1/1
  Trigonometric Function1/1 -> [Beta], Scope4/1
  [V_mag] -> Bus Creator/1  "V_mag"
  [Mach] -> Bus Creator/2  "Mach"
  [Alpha] -> Bus Creator/3  "alpha"
  [Beta] -> Bus Creator/4  "beta"
  Bus Creator/1 -> Flight_Performance/1
  Bus Selector2/2 -> [air_density]  "<air_density>"
  [V_mag] -> Math Function/1
  Math Function/1 -> Product4/1
  [air_density] -> Product4/2
  Product4/1 -> Gain/1
  Gain/1 -> [dynamic_pressure]
  [dynamic_pressure] -> Bus Creator/5  "dynamic_pressure"
  Gain2/1 -> Scope7/1

== system A320_Model_v1_4_3/Navigation/Gravity Model ==
  note: Somigliana denklemi uygulanmýþtýr. Noureldin-Karamat sf.53
  Latitude : Inport
  Altitude : Inport  Port=2
  Constant : Constant
  Constant2 : Constant  Value=somigliana_coeff_a2
  Constant3 : Constant  Value=somigliana_coeff_a3
  Constant4 : Constant  Value=somigliana_coeff_a1
  Constant5 : Constant  Value=somigliana_coeff_a4
  Constant6 : Constant  Value=somigliana_coeff_a5
  Constant7 : Constant  Value=somigliana_coeff_a6
  Product{,2,4..6} (5 alike) : Product  RndMeth=Zero
  Product3 : Product  Inputs=3  RndMeth=Zero
  Product7 : Product  Inputs=3  RndMeth=Zero
  Sum1 : Sum  Inputs=+++
  Sum2 : Sum  Inputs=+++
  Sum3 : Sum  Inputs=|++
  Trigonometric Function2 : Trigonometry
  Acc_gravity : Outport
  wires:
  Altitude/1 -> [Altitude]
  Latitude/1 -> Trigonometric Function2/1
  Product/1 -> [sL2]
  Trigonometric Function2/1 -> Product/1, Product/2
  Constant2/1 -> Product2/1
  [sL2] -> Product2/2
  [sL2] -> Product3/2, Product3/3
  Constant3/1 -> Product3/1
  Constant/1 -> Sum2/1
  Product2/1 -> Sum2/2
  Product3/1 -> Sum2/3
  Constant4/1 -> Product4/1
  Sum2/1 -> Product4/2
  Product4/1 -> Sum1/1
  Constant5/1 -> Sum3/1
  Constant6/1 -> Product5/1
  [sL2] -> Product5/2
  Product5/1 -> Sum3/2
  Sum3/1 -> Product6/1
  [Altitude] -> Product6/2
  Product6/1 -> Sum1/2
  Constant7/1 -> Product7/1
  [Altitude] -> Product7/2, Product7/3
  Product7/1 -> Sum1/3
  Sum1/1 -> [acc_grav]
  [acc_grav] -> Acc_gravity/1

== system A320_Model_v1_4_3/Navigation/Normal and Meridian Radii ==
  Latitude : Inport
  Constant : Constant
  Constant3 : Constant  Value=a_Earth
  Constant4 : Constant  Value=e_Earth
  Constant5 : Constant  Value=a_Earth
  Constant6 : Constant
  Constant7 : Constant  Value=e_Earth
  Constant8 : Constant  Value=3
  Math Function : Math  Operator=square  SaturateOnIntegerOverflow=on
  Math Function1 : Math  Operator=square  SaturateOnIntegerOverflow=on
  Math Function2 : Math  Operator=pow  SaturateOnIntegerOverflow=on
  Product2 : Product  Inputs=*/  RndMeth=Zero
  Product3 : Product  RndMeth=Zero
  Product6 : Product  RndMeth=Zero
  Product7 : Product  Inputs=/*  RndMeth=Zero
  Sqrt : Sqrt  SaturateOnIntegerOverflow=on
  Sum1 : Sum  Inputs=|+-
  Sum2 : Sum  Inputs=|+-
  Trigonometric Function1 : Trigonometry
  R_N : Outport
  R_M : Outport  Port=2
  wires:
  Latitude/1 -> Trigonometric Function1/1
  [RN] -> R_N/1  "normal_radius"
  Constant3/1 -> Product2/1
  Constant/1 -> Sum1/1
  Trigonometric Function1/1 -> [sin_L]
  Constant4/1 -> Product3/1
  [sin_L] -> Product3/2
  Product3/1 -> Math Function1/1
  Math Function1/1 -> Sum1/2
  Sum1/1 -> Sqrt/1
  Sqrt/1 -> Product2/2, Math Function2/1
  Product2/1 -> [RN]
  Constant6/1 -> Sum2/1
  Constant7/1 -> Math Function/1
  Math Function/1 -> Sum2/2
  Constant5/1 -> Product6/1
  Sum2/1 -> Product6/2
  Product6/1 -> Product7/2
  Constant8/1 -> Math Function2/2
  Math Function2/1 -> Product7/1
  Product7/1 -> [RM]
  [RM] -> R_M/1  "Meridian_radius"

== system A320_Model_v1_4_3/Navigation/Position Integration ==
  Vel_NED : Inport
  R_N : Inport  Port=2
  Add1 : Sum
  Add5 : Sum
  Bus Creator : BusCreator  Inputs=3
  Demux : Demux  Outputs=3
  Gain : Gain  Gain=-1
  Integrator : Integrator  InitialCondition=initial_mulh(1)*pi/180
  Integrator2 : Integrator  InitialCondition=initial_mulh(2)*pi/180
  Integrator3 : Integrator  InitialCondition=initial_mulh(3)
  Product1 : Product  Inputs=*/  RndMeth=Zero
  Product4 : Product  Inputs=*//  RndMeth=Zero
  Trigonometric Function : Trigonometry  Operator=cos
  mulh : Outport
  wires:
  Vel_NED/1 -> Demux/1
  Demux/1 -> [Vel_N]
  Demux/2 -> [Vel_E]
  Demux/3 -> [Vel_D]
  R_N/1 -> [R_N]
  [Vel_N] -> Product1/1
  [alt] -> Add1/1
  [R_N] -> Add1/2
  Add1/1 -> Product1/2
  Product1/1 -> Integrator/1
  [Vel_E] -> Product4/1
  [alt] -> Add5/1
  [R_N] -> Add5/2
  Add5/1 -> Product4/2
  Product4/1 -> Integrator2/1
  Integrator/1 -> [lat]
  [lat] -> Trigonometric Function/1
  Trigonometric Function/1 -> Product4/3
  Integrator2/1 -> [lon]
  [Vel_D] -> Gain/1
  Integrator3/1 -> [alt]
  [lat] -> Bus Creator/1  "latitude"
  [lon] -> Bus Creator/2  "longitude"
  [alt] -> Bus Creator/3  "altitude"
  Bus Creator/1 -> mulh/1  "mulh"
  Gain/1 -> Integrator3/1

== system A320_Model_v1_4_3/Navigation/Taken Distance ==
  Vel_NED : Inport
  Demux : Demux  Outputs=3
  Dot Product : DotProduct  InputSameDT=on  OutDataTypeStr=Inherit: Inherit via internal rule
  Integrator1 : Integrator
  Mux1 : Mux  Inputs=2
  Sqrt : Sqrt  SaturateOnIntegerOverflow=on
  Terminator : Terminator
  Taken_distance : Outport
  wires:
  [taken_distance] -> Taken_distance/1  "taken_distance"
  Demux/3 -> Terminator/1
  Demux/2 -> [Vel_E]
  Demux/1 -> [Vel_N]
  Vel_NED/1 -> Demux/1
  Dot Product/1 -> Sqrt/1
  Sqrt/1 -> Integrator1/1
  Mux1/1 -> Dot Product/1, Dot Product/2
  Integrator1/1 -> [taken_distance]
  [Vel_N] -> Mux1/1
  [Vel_E] -> Mux1/2

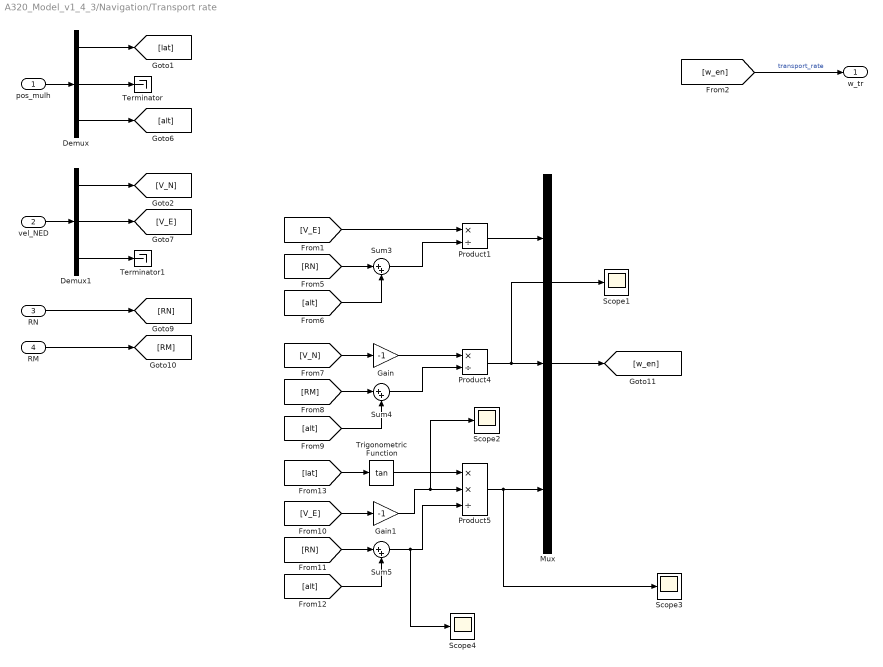
== system A320_Model_v1_4_3/Navigation/Transport rate ==
  pos_mulh : Inport
  vel_NED : Inport  Port=2
  RN : Inport  Port=3
  RM : Inport  Port=4
  Demux : Demux  Outputs=3
  Demux1 : Demux  Outputs=3
  Gain : Gain  Gain=-1
  Gain1 : Gain  Gain=-1
  Mux : Mux  Inputs=3
  Product1 : Product  Inputs=*/  RndMeth=Zero
  Product4 : Product  Inputs=*/  RndMeth=Zero
  Product5 : Product  Inputs=**/  RndMeth=Zero
  Scope{1..4} (4 alike) : Scope
  Sum3 : Sum  Inputs=|++
  Sum4 : Sum  Inputs=|++
  Sum5 : Sum  Inputs=|++
  Terminator : Terminator
  Terminator1 : Terminator
  Trigonometric Function : Trigonometry  Operator=tan
  w_tr : Outport
  wires:
  [w_en] -> w_tr/1  "transport_rate"
  Demux/1 -> [lat]
  Demux/2 -> Terminator/1
  Demux/3 -> [alt]
  vel_NED/1 -> Demux1/1
  Demux1/1 -> [V_N]
  Demux1/2 -> [V_E]
  Demux1/3 -> Terminator1/1
  pos_mulh/1 -> Demux/1
  RN/1 -> [RN]
  RM/1 -> [RM]
  [V_E] -> Product1/1
  [RN] -> Sum3/1
  [alt] -> Sum3/2
  Sum3/1 -> Product1/2
  [V_N] -> Gain/1
  [RM] -> Sum4/1
  [alt] -> Sum4/2
  Sum4/1 -> Product4/2
  Gain/1 -> Product4/1
  [V_E] -> Gain1/1
  [RN] -> Sum5/1
  [alt] -> Sum5/2
  [lat] -> Trigonometric Function/1
  Trigonometric Function/1 -> Product5/1
  Sum5/1 -> Product5/3, Scope4/1
  Gain1/1 -> Product5/2, Scope2/1
  Product1/1 -> Mux/1
  Product4/1 -> Mux/2, Scope1/1
  Product5/1 -> Mux/3, Scope3/1
  Mux/1 -> [w_en]

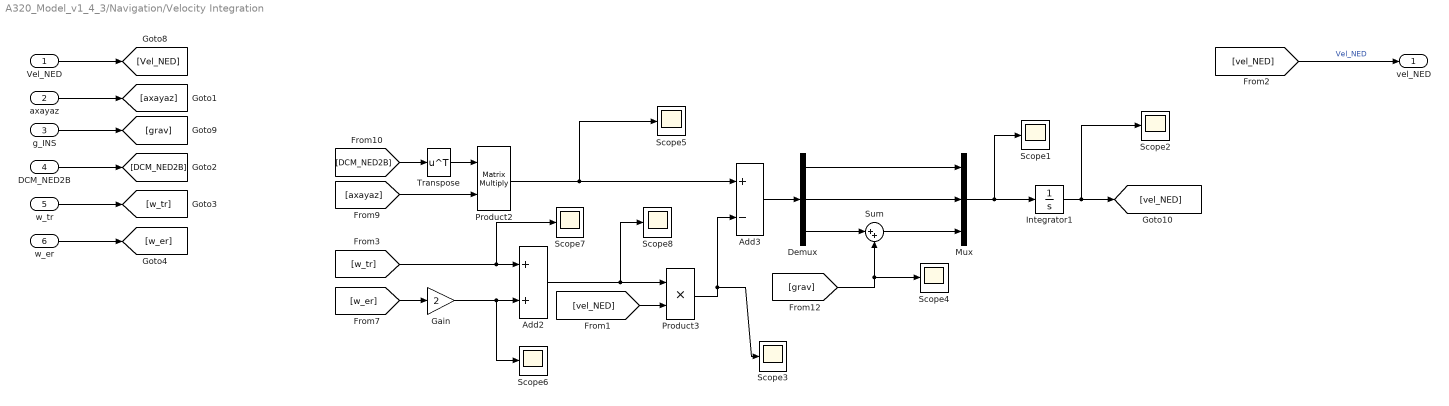
== system A320_Model_v1_4_3/Navigation/Velocity Integration ==
  Vel_NED : Inport
  axayaz : Inport  Port=2
  g_INS : Inport  Port=3
  DCM_NED2B : Inport  Port=4
  w_tr : Inport  Port=5
  w_er : Inport  Port=6
  Add2 : Sum
  Add3 : Sum  Inputs=+-
  Demux : Demux  Outputs=3
  Gain : Gain  Gain=2
  Integrator1 : Integrator  InitialCondition=initial_vel_NED
  Mux : Mux  Inputs=3
  Product2 : Product  Multiplication=Matrix(*)  RndMeth=Zero
  Product3 : Product  RndMeth=Zero
  Scope{1..8} (8 alike) : Scope
  Sum : Sum  Inputs=|++
  Transpose : Math  Operator=transpose  SaturateOnIntegerOverflow=on
  vel_NED : Outport
  wires:
  w_er/1 -> [w_er]
  w_tr/1 -> [w_tr]
  DCM_NED2B/1 -> [DCM_NED2B]
  [vel_NED] -> vel_NED/1  "Vel_NED"
  axayaz/1 -> [axayaz]
  Vel_NED/1 -> [Vel_NED]
  g_INS/1 -> [grav]
  [w_er] -> Gain/1
  [w_tr] -> Add2/1, Scope7/1
  Gain/1 -> Add2/2, Scope6/1
  [DCM_NED2B] -> Transpose/1
  [axayaz] -> Product2/2
  Add2/1 -> Product3/1, Scope8/1
  [vel_NED] -> Product3/2
  Product3/1 -> Add3/2, Scope3/1
  Mux/1 -> Integrator1/1, Scope1/1
  Integrator1/1 -> [vel_NED], Scope2/1
  Add3/1 -> Demux/1
  Demux/1 -> Mux/1
  Demux/2 -> Mux/2
  Demux/3 -> Sum/1
  Sum/1 -> Mux/3
  [grav] -> Sum/2, Scope4/1
  Transpose/1 -> Product2/1
  Product2/1 -> Add3/1, Scope5/1
